simulink model "cv03"  (R2024b)
settings: Solver=VariableStepAuto  StartTime=0.0  StopTime=400  RelTol=1e-3
undefined symbols (not defined in the file): m, n
settings Model: Creator=baron  LastModifiedBy=baron

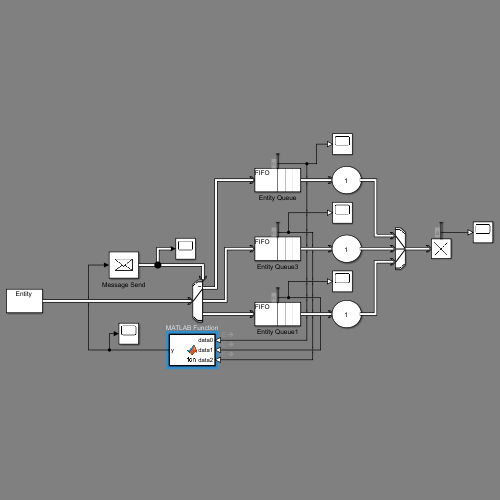
[thumbnail: Simulink's stored preview of the top-level diagram]
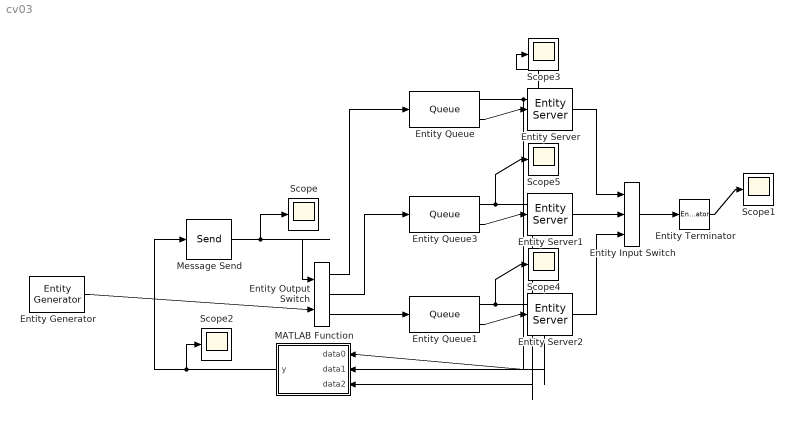
== system cv03 ==
  Entity Input Switch : EntityInputSwitch  InputPortMessageModes=m,m,m  OutputPortMessageModes=m  NumberInputPorts=3
      settings: InputPortMap=u1,u2,u3
  Entity Output Switch : EntityOutputSwitch  InputPortMessageModes=m,m  OutputPortMessageModes=m,m,m  NumberOutputPorts=3  SwitchingCriterion=From control port  SwitchAttributeName=Attribute1
      settings: InputPortMap=u0,u1  OutputPortMap=o0,o1,o2
  Entity Generator : EntityGenerator  OutputPortMessageModes=m  TimeSource=MATLAB action  IntergenerationTimeAction=|  AttributeName=timeWait  EntityType=Structured  EntityTypeName=Entity
      | persistent rngInit;
      | if isempty(rngInit)
      |     seed = 12345;
      |     rng(seed);
      |     rngInit = true;
      | end
      | 
      | % Pattern: Uniform distribution
      | % m: Minimum, M: Maximum
      | m = 0.1; M = 5;
      | dt = m + (M - m) * rand;
  Entity Queue : Queue  InputPortMessageModes=m  OutputPortMessageModes=n,m  Capacity=5  NumberEntitiesInBlock=on
      settings: OutputPortMap=o1,o5
  Entity Queue1 : Queue  InputPortMessageModes=m  OutputPortMessageModes=n,m  Capacity=5  NumberEntitiesInBlock=on
      settings: OutputPortMap=o1,o5
  Entity Queue3 : Queue  InputPortMessageModes=m  OutputPortMessageModes=n,m  Capacity=5  NumberEntitiesInBlock=on
      settings: OutputPortMap=o1,o5
  Entity Server : EntityServer  InputPortMessageModes=m  OutputPortMessageModes=m  Capacity=1  ServiceTimeSource=MATLAB action  ServiceTimeAttributeName=timeWait  ServiceTimeAction=|
      | persistent rngInit;
      | if isempty(rngInit)
      |     seed = 12345;
      |     rng(seed);
      |     rngInit = true;
      | end
      | 
      | % Pattern: Uniform distribution
      | % m: Minimum, M: Maximum
      | m = 5; M = 15;
      | dt = m + (M - m) * rand;
  Entity Server1 : EntityServer  InputPortMessageModes=m  OutputPortMessageModes=m  Capacity=1  ServiceTimeSource=MATLAB action  ServiceTimeAttributeName=timeWait  ServiceTimeAction=|
      | persistent rngInit;
      | if isempty(rngInit)
      |     seed = 12345;
      |     rng(seed);
      |     rngInit = true;
      | end
      | 
      | % Pattern: Uniform distribution
      | % m: Minimum, M: Maximum
      | m = 5; M = 15;
      | dt = m + (M - m) * rand;
  Entity Server2 : EntityServer  InputPortMessageModes=m  OutputPortMessageModes=m  Capacity=1  ServiceTimeSource=MATLAB action  ServiceTimeAttributeName=timeWait  ServiceTimeAction=|
      | persistent rngInit;
      | if isempty(rngInit)
      |     seed = 12345;
      |     rng(seed);
      |     rngInit = true;
      | end
      | 
      | % Pattern: Uniform distribution
      | % m: Minimum, M: Maximum
      | m = 5; M = 15;
      | dt = m + (M - m) * rand;
  Entity Terminator : EntityTerminator  InputPortMessageModes=m  NumberEntitiesArrived=on
      settings: OutputPortMap=o0
  MATLAB Function : MATLAB Function  TreatAsAtomicUnit=on
  Message Send : Send  OutputPortMessageModes=m
  Scope{,1..5} (6 alike) : Scope
  wires:
  Message Send/1 -> Entity Output Switch/1, Scope/1
  Entity Queue/2 -> Entity Server/1
  Entity Queue/1 -> MATLAB Function/1(data0), Scope3/1
  Entity Output Switch/2 -> Entity Queue3/1
  Entity Generator/1 -> Entity Output Switch/2
  MATLAB Function/1(y) -> Message Send/1, Scope2/1
  Entity Output Switch/1 -> Entity Queue/1
  Entity Output Switch/3 -> Entity Queue1/1
  Entity Queue3/2 -> Entity Server1/1
  Entity Queue3/1 -> MATLAB Function/3(data2), Scope5/1
  Entity Queue1/2 -> Entity Server2/1
  Entity Queue1/1 -> MATLAB Function/2(data1), Scope4/1
  Entity Server/1 -> Entity Input Switch/1
  Entity Server1/1 -> Entity Input Switch/2
  Entity Server2/1 -> Entity Input Switch/3
  Entity Input Switch/1 -> Entity Terminator/1
  Entity Terminator/1 -> Scope1/1

== matlab function cv03/MATLAB Function ==
  data: data0 input; data1 input; y output; data2 input
function y = fcn(data0, data1, data2)

[~,y] = min([data0 data1 data2]);
end
